simulink model "Batterie_Converter"  (R2024a)
settings: Solver=FixedStepAuto  StartTime=0.0  StopTime=4  FixedStep=1e-6  RelTol=1e-3
values from neighbouring files (symbols this model uses):
  C_Bat = 1e-3    (= 0.001)    [Parameters.m]    (also in Params_Battery_converter.m)
  ki_Ibat = 550    [Parameters.m]    (also in Params_Battery_converter.m)
  ki_Vbat = 20    [Parameters.m]    (also in Params_Battery_converter.m)
  kp_Ibat = 6.28    [Parameters.m]    (also in Params_Battery_converter.m)
  kp_Vbat = 0.2    [Parameters.m]    (also in Params_Battery_converter.m)
  L_Bat = 2e-3    (= 0.002)    [Parameters.m]    (also in Params_Battery_converter.m)
  R_ch = 49    [Params_Battery_converter.m]
undefined symbols (not defined in the file or in its folder): Cap_exp_Bat, Ion, Lithium, R_int, V_exp_Bat
libraries: spsSeriesRLCBranchLib x4, spsIdealSwitchLib x4, spsCurrentMeasurementLib x3, spsBatteryLib x2, slpidlib x2, spsIGBTDiodeLib x2, spsVoltageMeasurementLib x2, spsPWMGenerator2LevelLib x1, spsDCVoltageSourceLib x1, spspowerguiLib x1
settings Model: Creator=K Edd Edd  LastModifiedBy=K Edd Edd

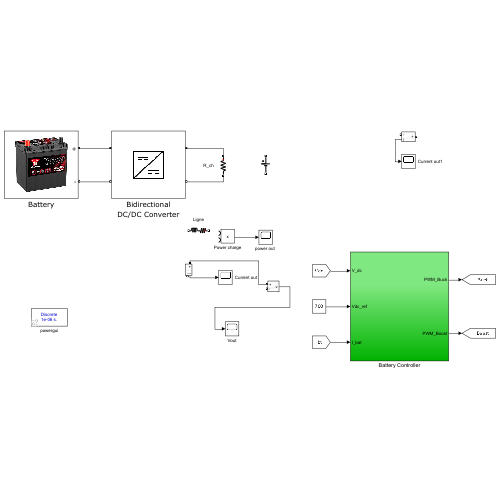
[thumbnail: Simulink's stored preview of the top-level diagram]
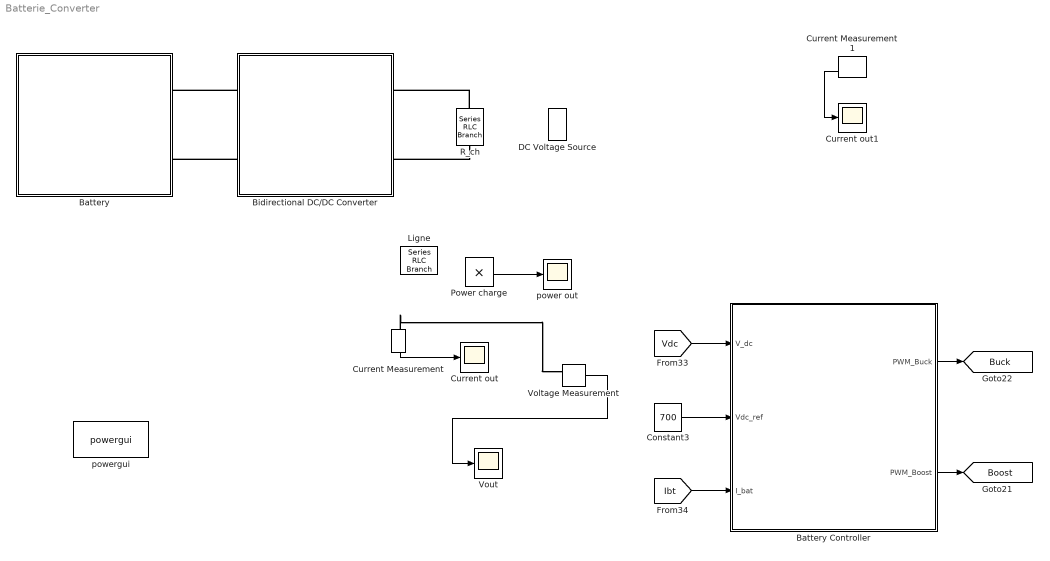
== system Batterie_Converter ==
  Battery : Subsystem
      mask Display: image('Batterie.jpg');
  Battery Controller : Subsystem
  Bidirectional DC/DC Converter : Subsystem
      mask Display: image('CC-CC-converter.png');
  Constant3 : Constant  Value=700
  Current Measurement : spsCurrentMeasurementLib/Current Measurement  PhasorSimulation=off  OutputType=Complex  PSBequivalent=0
  Current Measurement1 : spsCurrentMeasurementLib/Current Measurement  PhasorSimulation=off  OutputType=Complex  PSBequivalent=0
  Current out : Scope
  Current out1 : Scope
  DC Voltage Source : spsDCVoltageSourceLib/DC Voltage Source  Amplitude=700  Measurements=None
  Ligne : spsSeriesRLCBranchLib/Series RLC Branch  LConnTagsString=__new0  RConnTagsString=__new0  BranchType=RL  Resistance=0.1  Inductance=1e-5  SetiL0=off  InitialCurrent=0  Capacitance=1e-6  Setx0=off  InitialVoltage=0  Measurements=None
  Power charge : Product
  R_ch : spsSeriesRLCBranchLib/Series RLC Branch  LConnTagsString=__new0  RConnTagsString=__new0  BranchType=R  Resistance=R_ch  Inductance=1e-3  SetiL0=off  InitialCurrent=0  Capacitance=1e-6  Setx0=off  InitialVoltage=0  Measurements=None
  Voltage Measurement : spsVoltageMeasurementLib/Voltage Measurement  PhasorSimulation=off  OutputType=Complex  PSBequivalent=0
  Vout : Scope
  "power out " : Scope
  powergui : spspowerguiLib/powergui  Priority=1  SimulationMode=Discrete  SampleTime=1e-6  frequency=60  Iterations=50  frequencyindice=0  Pbase=100e6  ErrMax=1e-4  UnitsV=kV  UnitsW=MW  buscounter=0  FunctionMessages=off  echomessages=off  EnableUseOfTLC=off  CurrentSourceSwitches=off  DisableSnubberDevices=off  DisableRonSwitches=off  DisableVfSwitches=off  DisplayEquations=off  AutomaticDiscreteSolvers=off  SolverType=Tustin/Backward Euler (TBE)  Interpol=off  ExternalGateDelay=off  methode=off  Ts=100  x0status=blocks  SPID=on  SwTol=0  HookPort=off  NonlinearTolerance=1e-4  nMaxIteration=100  ContinueOnMaxIteration=off  RestoreLinks=warning  ResistiveCurrentMeasurement=off  Frange=[0:2:500]  Ylog=off  Xlog=on  ShowGrid=off  save=off  variable=ZData  structure=0  ZoomFFT=off  StartTime=0.0  cycles=1  DisplayStyle=1  fundamental=60  FreqAxis=off  MaxFrequency=1000  frequencyindicesteady=1  RmsSteady=1  display=off
  tag scope: Boost=global, Buck=global
  wires:
  Battery Controller/2(PWM_Boost) -> [Boost]
  [Vdc] -> Battery Controller/1(V_dc)
  Battery Controller/1(PWM_Buck) -> [Buck]
  [Ibt] -> Battery Controller/3(I_bat)
  Constant3/1 -> Battery Controller/2(Vdc_ref)
  Voltage Measurement/1 -> Vout/1
  Current Measurement/1 -> Current out/1
  Power charge/1 -> "power out "/1
  Current Measurement1/1 -> Current out1/1
  connections:
  Bidirectional DC/DC Converter/RConn2 -- Battery/LConn2
  Bidirectional DC/DC Converter/RConn1 -- Battery/LConn1
  R_ch/RConn1 -- Bidirectional DC/DC Converter/LConn2
  Current Measurement/LConn1 -- Voltage Measurement/LConn1
  R_ch/LConn1 -- Bidirectional DC/DC Converter/LConn1

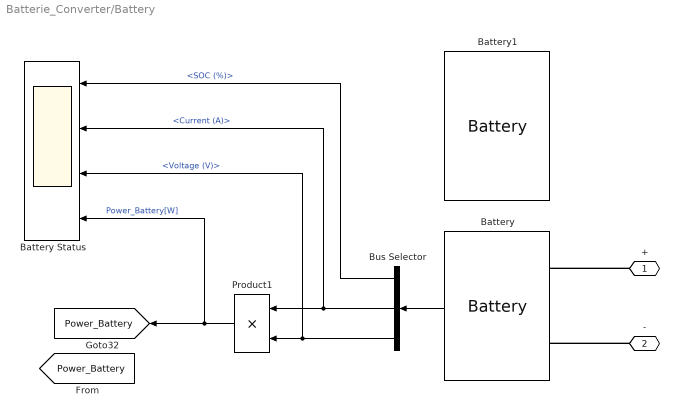
== system Batterie_Converter/Battery ==
  Battery : spsBatteryLib/Battery  BatType=Lithium-Ion  ShowTempParam=off  ThermalPreset=no  ShowAgeParam=off  NomV=500  NomQ=100  SOC=90  Batt_Tr=0.01  PresetModel=off  MaxQ=40  MinV=V_cut  FullV=V_full  Dis_rate=I_nom_dis  R=R_int  Normal_OP=Cap_Vnom_Bat  expZone="[V_exp_Bat      Cap_exp_Bat]"  current=[1.5 3]  Units=Ampere-hour  Tci=20  NomT=25  T2=0  MaxQ2=2.208  FullV2=3.45  Normal_OP2=2.8  expZone2="[3.22        0.23]"  Rca=0.6  ti=1000  Dp=0  Neq0=0  Tsim=1e6  Ta1=25  Qeol=5.4*0.9  Reol=0.013333*1.2  Char_age=[2.3478, 3]  Dis_age=[2.3478, 10]  N1=1500  N2=10500  N3=1000  N4=1400  Ta2=45  N5=950
      settings: LibrarySourceBlock=electricdrivelib/Extra Sources/Battery
  Battery Status : Scope  NumInputPorts=4
  Battery1 : spsBatteryLib/Battery  BatType=Lithium-Ion  ShowTempParam=off  ThermalPreset=no  ShowAgeParam=off  NomV=V_nom  NomQ=Cap_nom  SOC=SOC_init  Batt_Tr=T_resp  PresetModel=off  MaxQ=40  MinV=V_cut  FullV=V_full  Dis_rate=I_nom_dis  R=R_int  Normal_OP=Cap_Vnom_Bat  expZone="[V_exp_Bat      Cap_exp_Bat]"  current=[1.5 3]  Units=Ampere-hour  Tci=20  NomT=25  T2=0  MaxQ2=2.208  FullV2=3.45  Normal_OP2=2.8  expZone2="[3.22        0.23]"  Rca=0.6  ti=1000  Dp=0  Neq0=0  Tsim=1e6  Ta1=25  Qeol=5.4*0.9  Reol=0.013333*1.2  Char_age=[2.3478, 3]  Dis_age=[2.3478, 10]  N1=1500  N2=10500  N3=1000  N4=1400  Ta2=45  N5=950
      settings: LibrarySourceBlock=electricdrivelib/Extra Sources/Battery
  Bus Selector : BusSelector  OutputSignals=SOC (%),Current (A),Voltage (V)
  Product1 : Product  RndMeth=Zero
  + : PMIOPort  Side=Left
  - : PMIOPort  Port=2  Side=Left
  tag scope: Power_Battery=global
  wires:
  Product1/1 -> [Power_Battery], Battery Status/4  "Power_Battery[W]"
  Bus Selector/1 -> Battery Status/1  "<SOC (%)>"
  Bus Selector/3 -> Product1/2, Battery Status/3  "<Voltage (V)>"
  Battery/1 -> Bus Selector/1
  Bus Selector/2 -> Product1/1, Battery Status/2  "<Current (A)>"
  connections:
  +/RConn1 -- Battery/LConn1
  -/RConn1 -- Battery/LConn2

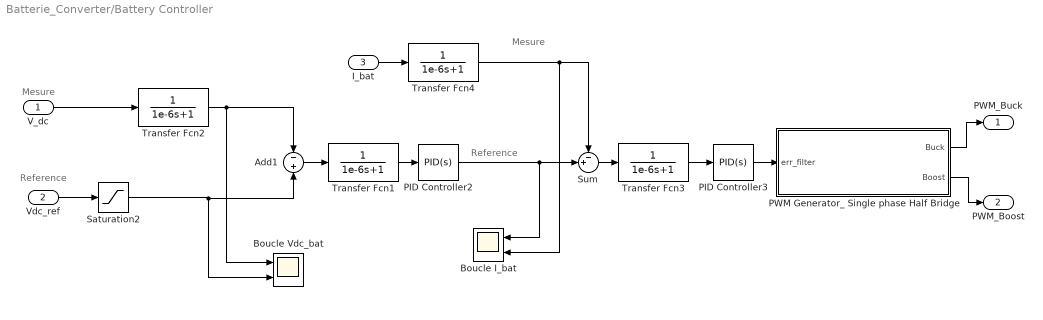
== system Batterie_Converter/Battery Controller ==
  note: Mesure
  note: Reference
  note: Mesure
  note: Reference
  V_dc : Inport
  Vdc_ref : Inport  Port=2
  I_bat : Inport  Port=3
  Add1 : Sum  Inputs=-+
  Boucle I_bat : Scope  NumInputPorts=2
  Boucle Vdc_bat : Scope  NumInputPorts=2
  PID Controller2 : slpidlib/PID Controller  Controller=PID  Form=Parallel  TimeDomain=Continuous-time  UseExternalTs=off  SampleTime=-1  IntegratorMethod=Forward Euler  FilterMethod=Forward Euler  ControllerParametersSource=internal  P=kp_Vbat  I=ki_Vbat  UseKiTs=off  D=0  UseExternalDerivativeSource=off  N=100  UseFilter=on  TunerSelectOption=Transfer Function Based (PID Tuner App)  InitialConditionSource=internal  InitialConditionForIntegrator=0  InitialConditionForFilter=0  DifferentiatorICPrevScaledInput=0  ExternalReset=none  TrackingMode=off  Kt=1  LimitOutput=off  SatLimitsSource=internal  UpperSaturationLimit=inf  LowerSaturationLimit=-inf  LinearizeAsGain=off  AntiWindupMode=none  Kb=1  LimitIntegrator=off  UpperIntegratorSaturationLimit=inf  LowerIntegratorSaturationLimit=-inf  POutMin=[]  POutMax=[]  IOutMin=[]  IOutMax=[]  DOutMin=[]  DOutMax=[]  NOutMin=[]  NOutMax=[]  SumOutMin=[]  SumOutMax=[]  SaturationOutMin=[]  SaturationOutMax=[]  PParamMin=[]  PParamMax=[]  IParamMin=[]  IParamMax=[]  DParamMin=[]  DParamMax=[]  NParamMin=[]  NParamMax=[]  KbParamMin=[]  KbParamMax=[]  KtParamMin=[]  KtParamMax=[]  KbOutMin=[]  KbOutMax=[]  KtOutMin=[]  KtOutMax=[]  IntegratorOutMin=[]  IntegratorOutMax=[]  FilterOutMin=[]  FilterOutMax=[]  SumI1OutMin=[]  SumI1OutMax=[]  SumI2OutMin=[]  SumI2OutMax=[]  SumI3OutMin=[]  SumI3OutMax=[]  SumI4OutMin=[]  SumI4OutMax=[]  SumDOutMin=[]  SumDOutMax=[]  DifferentiatorOutMin=[]  DifferentiatorOutMax=[]  FilterDiffOutCoefMin=[]  FilterDiffOutCoefMax=[]  ReciprocalOutMin=[]  ReciprocalOutMax=[]  SumDenOutMin=[]  SumDenOutMax=[]  SumNumOutMin=[]  SumNumOutMax=[]  DivideOutMin=[]  DivideOutMax=[]  UdiffTsProdOutMin=[]  UdiffTsProdOutMax=[]  NTsProdOutMin=[]  NTsProdOutMax=[]  UintegralTsProdOutMin=[]  UintegralTsProdOutMax=[]  UngainTsProdOutMin=[]  UngainTsProdOutMax=[]  ClampingZeroOutDataTypeStr=Inherit: Inherit via back propagation  ClampingZeroOutMin=[]  ClampingZeroOutMax=[]  FilterDenConstantOutDataTypeStr=Inherit: Inherit via back propagation  FilterDenConstantOutMin=[]  FilterDenConstantOutMax=[]  PCopyOutDataTypeStr=Inherit: Inherit via back propagation  PCopyOutMin=[]  PCopyOutMax=[]  NCopyOutDataTypeStr=Inherit: Inherit via back propagation  NCopyOutMin=[]  NCopyOutMax=[]  IntegratorContinuousStateAttributes=''  IntegratorStateMustResolveToSignalObject=off  IntegratorRTWStateStorageClass=Auto  FilterContinuousStateAttributes=''  FilterStateMustResolveToSignalObject=off  FilterRTWStateStorageClass=Auto  ParallelPVariant=InternalParameters  IdealPVariant=Disabled  IVariant=InternalParameters  DVariant=InternalParameters  IntegratorVariant=Continuous  SatVariant=Disabled  AWVariant=Passthrough  PCopyVariant=Disabled  TRVariant=Disabled  FdbkBlocksVariant=Forward  IdealPFdbkVariant=Disabled  SatFdbkVariant=Disabled  DerivativeFilterVariant=ContFilter  NVariant=InternalParameters  NCopyVariant=Disabled  FilterICVariant=InternalICsFilter  IntegratorICVariant=InternalICs  ExternalResetVariant=Disabled  TRSumVariant=Passthrough  SumFdbkVariant=Disabled  SumVariant=Sum_PID  TsampFilterVariant=InternalTs  TsampNgainVariant=Passthrough  TsampIntegralVariant=Disabled_SignalSpec  ExternalSaturationOutDataTypeStr=Inherit: Same as second input  DerivativeSourceVariant=ErrorSignal
  PID Controller3 : slpidlib/PID Controller  Controller=PID  Form=Parallel  TimeDomain=Continuous-time  UseExternalTs=off  SampleTime=-1  IntegratorMethod=Forward Euler  FilterMethod=Forward Euler  ControllerParametersSource=internal  P=kp_Ibat  I=ki_Ibat  UseKiTs=off  D=0  UseExternalDerivativeSource=off  N=100  UseFilter=on  TunerSelectOption=Transfer Function Based (PID Tuner App)  InitialConditionSource=internal  InitialConditionForIntegrator=0  InitialConditionForFilter=0  DifferentiatorICPrevScaledInput=0  ExternalReset=none  TrackingMode=off  Kt=1  LimitOutput=off  SatLimitsSource=internal  UpperSaturationLimit=inf  LowerSaturationLimit=-inf  LinearizeAsGain=off  AntiWindupMode=none  Kb=1  LimitIntegrator=off  UpperIntegratorSaturationLimit=inf  LowerIntegratorSaturationLimit=-inf  POutMin=[]  POutMax=[]  IOutMin=[]  IOutMax=[]  DOutMin=[]  DOutMax=[]  NOutMin=[]  NOutMax=[]  SumOutMin=[]  SumOutMax=[]  SaturationOutMin=[]  SaturationOutMax=[]  PParamMin=[]  PParamMax=[]  IParamMin=[]  IParamMax=[]  DParamMin=[]  DParamMax=[]  NParamMin=[]  NParamMax=[]  KbParamMin=[]  KbParamMax=[]  KtParamMin=[]  KtParamMax=[]  KbOutMin=[]  KbOutMax=[]  KtOutMin=[]  KtOutMax=[]  IntegratorOutMin=[]  IntegratorOutMax=[]  FilterOutMin=[]  FilterOutMax=[]  SumI1OutMin=[]  SumI1OutMax=[]  SumI2OutMin=[]  SumI2OutMax=[]  SumI3OutMin=[]  SumI3OutMax=[]  SumI4OutMin=[]  SumI4OutMax=[]  SumDOutMin=[]  SumDOutMax=[]  DifferentiatorOutMin=[]  DifferentiatorOutMax=[]  FilterDiffOutCoefMin=[]  FilterDiffOutCoefMax=[]  ReciprocalOutMin=[]  ReciprocalOutMax=[]  SumDenOutMin=[]  SumDenOutMax=[]  SumNumOutMin=[]  SumNumOutMax=[]  DivideOutMin=[]  DivideOutMax=[]  UdiffTsProdOutMin=[]  UdiffTsProdOutMax=[]  NTsProdOutMin=[]  NTsProdOutMax=[]  UintegralTsProdOutMin=[]  UintegralTsProdOutMax=[]  UngainTsProdOutMin=[]  UngainTsProdOutMax=[]  ClampingZeroOutDataTypeStr=Inherit: Inherit via back propagation  ClampingZeroOutMin=[]  ClampingZeroOutMax=[]  FilterDenConstantOutDataTypeStr=Inherit: Inherit via back propagation  FilterDenConstantOutMin=[]  FilterDenConstantOutMax=[]  PCopyOutDataTypeStr=Inherit: Inherit via back propagation  PCopyOutMin=[]  PCopyOutMax=[]  NCopyOutDataTypeStr=Inherit: Inherit via back propagation  NCopyOutMin=[]  NCopyOutMax=[]  IntegratorContinuousStateAttributes=''  IntegratorStateMustResolveToSignalObject=off  IntegratorRTWStateStorageClass=Auto  FilterContinuousStateAttributes=''  FilterStateMustResolveToSignalObject=off  FilterRTWStateStorageClass=Auto  ParallelPVariant=InternalParameters  IdealPVariant=Disabled  IVariant=InternalParameters  DVariant=InternalParameters  IntegratorVariant=Continuous  SatVariant=Disabled  AWVariant=Passthrough  PCopyVariant=Disabled  TRVariant=Disabled  FdbkBlocksVariant=Forward  IdealPFdbkVariant=Disabled  SatFdbkVariant=Disabled  DerivativeFilterVariant=ContFilter  NVariant=InternalParameters  NCopyVariant=Disabled  FilterICVariant=InternalICsFilter  IntegratorICVariant=InternalICs  ExternalResetVariant=Disabled  TRSumVariant=Passthrough  SumFdbkVariant=Disabled  SumVariant=Sum_PID  TsampFilterVariant=InternalTs  TsampNgainVariant=Passthrough  TsampIntegralVariant=Disabled_SignalSpec  ExternalSaturationOutDataTypeStr=Inherit: Same as second input  DerivativeSourceVariant=ErrorSignal
  PWM Generator_ Single phase Half Bridge : Subsystem
  Saturation2 : Saturate  UpperLimit=700  LowerLimit=0
  Sum : Sum  Inputs=-+|
  Transfer Fcn{1..4} (4 alike) : TransferFcn  Denominator=[1e-6 1]
  PWM_Buck : Outport  OutputWhenDisabled=reset  InitialOutput=0  VectorParamsAs1DForOutWhenUnconnected=off
  PWM_Boost : Outport  Port=2  OutputWhenDisabled=reset  InitialOutput=0  VectorParamsAs1DForOutWhenUnconnected=off
  wires:
  I_bat/1 -> Transfer Fcn4/1
  PWM Generator_ Single phase Half Bridge/1(Buck) -> PWM_Buck/1
  PWM Generator_ Single phase Half Bridge/2(Boost) -> PWM_Boost/1
  Vdc_ref/1 -> Saturation2/1
  PID Controller3/1 -> PWM Generator_ Single phase Half Bridge/1(err_filter)
  Add1/1 -> Transfer Fcn1/1
  Sum/1 -> Transfer Fcn3/1
  PID Controller2/1 -> Boucle I_bat/1, Sum/2
  Transfer Fcn2/1 -> Add1/1, Boucle Vdc_bat/1
  Transfer Fcn1/1 -> PID Controller2/1
  Transfer Fcn3/1 -> PID Controller3/1
  Transfer Fcn4/1 -> Boucle I_bat/2, Sum/1
  V_dc/1 -> Transfer Fcn2/1
  Saturation2/1 -> Boucle Vdc_bat/2, Add1/2

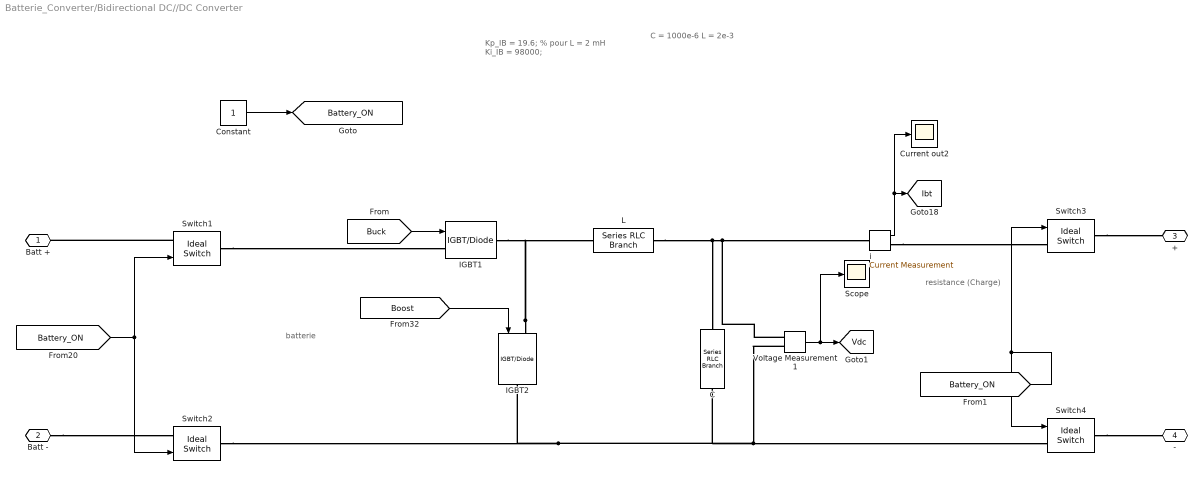
== system Batterie_Converter/Bidirectional DC//DC Converter ==
  note: batterie
  note: C = 1000e-6
      | L = 2e-3
  note: Kp_IB = 19.6;   % pour L = 2 mH
      | Ki_IB = 98000;
  note: resistance
      | (Charge)
  C : spsSeriesRLCBranchLib/Series RLC Branch  LConnTagsString=__new0  RConnTagsString=__new0  BranchType=C  Resistance=1  Inductance=1e-3  SetiL0=off  InitialCurrent=0  Capacitance=C_Bat  Setx0=on  InitialVoltage=700  Measurements=None
  Constant : Constant
  Current out2 : Scope
  IGBT1 : spsIGBTDiodeLib/IGBT//Diode  Ron=1e-3  Rs=1e5  Cs=inf  Measurements=off
  IGBT2 : spsIGBTDiodeLib/IGBT//Diode  Ron=1e-3  Rs=1e5  Cs=inf  Measurements=off
  L : spsSeriesRLCBranchLib/Series RLC Branch  LConnTagsString=__new0  RConnTagsString=__new0  BranchType=L  Resistance=1  Inductance=L_Bat  SetiL0=off  InitialCurrent=0  Capacitance=1000e-6  Setx0=off  InitialVoltage=0  Measurements=None
  Scope : Scope
  Switch{1..4} (4 alike) : spsIdealSwitchLib/Ideal Switch  Ron=0.001  Lon=0  IC=0  Rs=1e6  Cs=inf  Measurements=off
  Voltage Measurement1 : spsVoltageMeasurementLib/Voltage Measurement  PhasorSimulation=off  OutputType=Complex  PSBequivalent=0
  i : spsCurrentMeasurementLib/Current Measurement  PhasorSimulation=off  OutputType=Complex  PSBequivalent=0
  Batt + : PMIOPort  Side=Left
  Batt - : PMIOPort  Port=2  Side=Left
  + : PMIOPort  Port=3  Side=Right
  - : PMIOPort  Port=4  Side=Right
  tag scope: Battery_ON=global, Ibt=global, Vdc=global
  wires:
  [Boost] -> IGBT2/1
  [Buck] -> IGBT1/1
  i/1 -> Current out2/1, [Ibt]
  [Battery_ON] -> Switch3/1, Switch4/1
  [Battery_ON] -> Switch1/1, Switch2/1
  Constant/1 -> [Battery_ON]
  Voltage Measurement1/1 -> Scope/1, [Vdc]
  connections:
  IGBT2/LConn1 -- L/RConn1 -- IGBT1/RConn1
  L/LConn1 -- Voltage Measurement1/LConn1 -- i/LConn1 -- C/LConn1
  i/RConn1 -- Switch3/LConn1
  Switch3/RConn1 -- +/RConn1
  Switch4/RConn1 -- -/RConn1
  Switch1/RConn1 -- IGBT1/LConn1
  C/RConn1 -- IGBT2/RConn1 -- Switch2/RConn1 -- Voltage Measurement1/LConn2 -- Switch4/LConn1
  Batt -/RConn1 -- Switch2/LConn1
  Switch1/LConn1 -- Batt +/RConn1

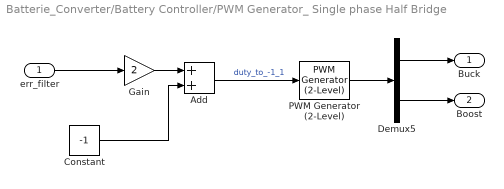
== system Batterie_Converter/Battery Controller/PWM Generator_ Single phase Half Bridge ==
  err_filter : Inport
  Add : Sum
  Constant : Constant  Value=-1
  Demux5 : Demux  Outputs=2
  Gain : Gain  Gain=2
  PWM Generator (2-Level) : spsPWMGenerator2LevelLib/PWM Generator (2-Level)  ModulatorType=Single-phase half-bridge (2 pulses)  ModulatorMode=Unsynchronized  Fc=Fc  Pc=90  nF=27  MinMax="[ -1  1 ]"  SamplingTechnique=Natural  ModulatingSignals=off  m=0.8  Freq=60  Phase=0  Ts=0  ShowCarrierOutport=off
  Buck : Outport
  Boost : Outport  Port=2
  wires:
  Constant/1 -> Add/2
  Gain/1 -> Add/1
  Demux5/2 -> Boost/1
  Add/1 -> PWM Generator (2-Level)/1  "duty_to_-1_1"
  err_filter/1 -> Gain/1
  Demux5/1 -> Buck/1
  PWM Generator (2-Level)/1 -> Demux5/1
